simulink model "test"  (R2023b)
settings: Solver=VariableStepAuto  StartTime=0.0  StopTime=inf  RelTol=1e-3
values from neighbouring files (symbols this model uses):
  A = [0  1; 0  0]    [1-dof.mat]    (also in 2-dof.mat = [0 0 0 0 1 0 0 0 0 0 0 0 ... (16 elements, 4x4)]; ball_balancing_platform.mat = [0 0 0 0 0 0 0 0 0 0 0 0 ... (64 elements, 8x8)])
  B = [0 -0.1692]    [1-dof.mat]    (also in 2-dof.mat = [0  0; -0.253868468945  0; 0  0; 0  0.253868468945]; ball_balancing_platform.mat = [0 0 0 0 0 0 1 0 0 0 0 0 ... (16 elements, 8x2)])
  C = [1 0]    [1-dof.mat]    (also in 2-dof.mat = [1  0  0  0; 0  0  1  0]; ball_balancing_platform.mat = [1 0 0 0 0 1 0 0 0 0 1 0 ... (32 elements, 4x8)])
  D = 0    [1-dof.mat]    (also in 2-dof.mat = [0  0; 0  0]; ball_balancing_platform.mat = [0  0; 0  0; 0  0; 0  0])
libraries: mpclib x1, aerolibanimutils x1
settings Model: Creator=farhan  LastModifiedBy=farhan

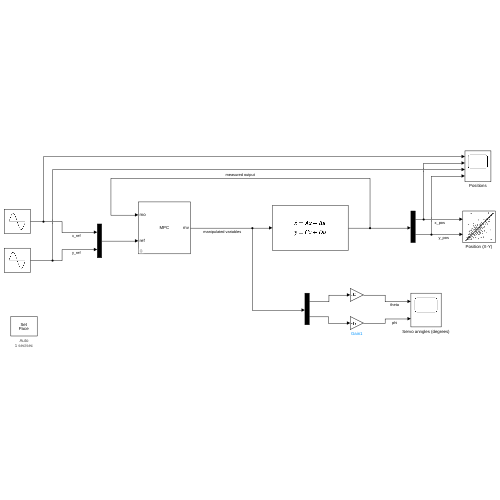
[thumbnail: Simulink's stored preview of the top-level diagram]
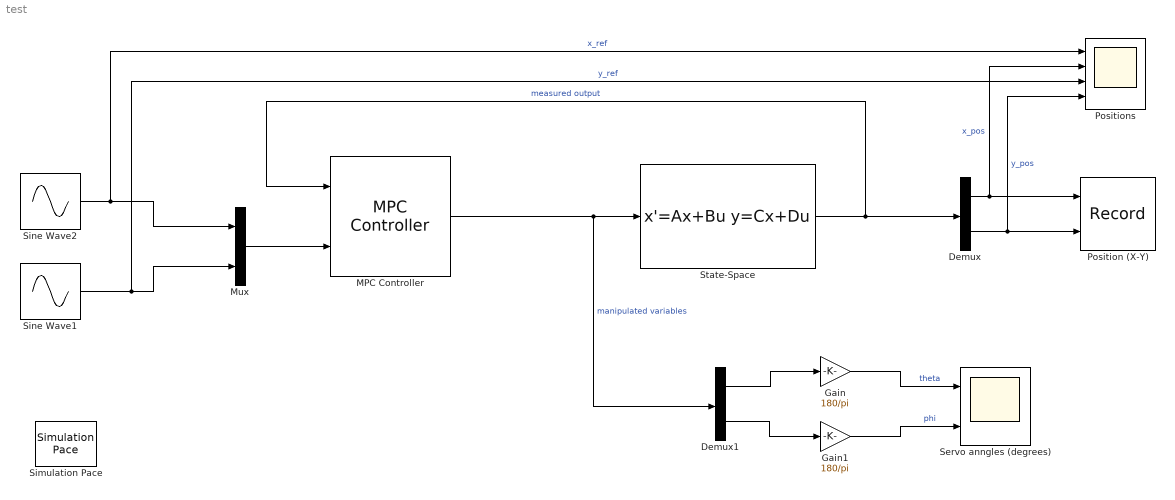
== system test ==
  Demux : Demux  Outputs=2
  Demux1 : Demux  Outputs=2
  Gain : Gain  Gain=180/pi
  Gain1 : Gain  Gain=180/pi
  MPC Controller : mpclib/MPC Controller  SCDEnableBlockLinearizationSpecification=on  mpcobj=mpc1  is_multiple=0  enable_value=0  return_u0=off  updateMPCinCallerWorkspace=on  md_inport=off  mv_inport=off  uref_inport=off  return_cost=off  return_mvseq=off  return_qpstatus=off  return_xseq=off  return_state=off  return_ovseq=off  state_inport=off  umin_inport=off  umax_inport=off  ymin_inport=off  ymax_inport=off  cc_inport=off  ywt_inport=off  uwt_inport=off  duwt_inport=off  rhoeps_inport=off  pm_inport=off  MaximumP=10  HorizonChoice=FixedHorizon  n_ts=0.1  n_p=7  n_mv=2  n_md=0  n_ud=0  n_mo=2  n_uo=0  BlockDataType=double  SampleTimeInherited=off  switch_inport=off
  Mux : Mux  Inputs=2
  Position (X-Y) : Record  FileSettingsInternal="{\"entries\":[{\"content\":{\"excelSettings\":{\"content\":{},\"type\":\"Streamout.ExcelSettings\"}},\"type\":\"Streamout.FileSettingStorage\",\"uuid\":\"\"}],\"packageUris\":[\"http:\\/\\/schema.mathworks.com\\/mf0\\/streamout_blocks\\/R2020a\"],\"version\":\"1.0\"}"  Layout=[1 1]  SignalsInternal="{\"entries\":[{\"content\":{\"signals\":[{\"content\":{\"blockPath\":[],\"dimensions\":[1],\"domain\":\"\",\"lineColor\":\"#fe330a\",\"port\":1,\"sid\":[\"\"],\"signalID\":130,\"signalName\":\"x_pos\"},\"type\":\"RecordBlkView.Signal\",\"uuid\":\"\"},{\"content\":{\"blockPath\":[],\"dimensions\":[1],\"domain\":\"\",\"lineColor\":\"#22b573\",\"port\":2,\"sid\":[\"\"],\"signalID\":134,\"signalName\":\"y_pos\"},\"type\":\"RecordBlkView.Signal\",\"uuid\":\"\"}]},\"type\":\"RecordBlkView.InputSignals\",\"uuid\":\"\"}],\"packageUris\":[\"http:\\/\\/schema.mathworks.com\\/mf0\\/streamout_blocks\\/R2020a\"],\"version\":\"1.0\"}"  VisualizationBindings="{\"xyplotplugin\":{\"info\":[{\"series\":[],\"subplotID\":1}]}}"  CompatibilityTag=XY
  Positions : Scope  NumInputPorts=4
  Servo anngles (degrees) : Scope  NumInputPorts=2
  Simulation Pace : aerolibanimutils/Simulation Pace  SimulationPace=1  SleepMode=Auto  OutputPaceError=off  SampleTime=1/30
  Sine Wave1 : Sin  Amplitude=0.15  Frequency=1.2  Phase=pi/2  SampleTime=0
  Sine Wave2 : Sin  Amplitude=0.15  Frequency=1.2  SampleTime=0
  State-Space : StateSpace  A=A  B=B  C=C  D=D  InitialCondition=0
  wires:
  MPC Controller/1 -> Demux1/1, State-Space/1  "manipulated variables"
  Mux/1 -> MPC Controller/2
  Sine Wave2/1 -> Mux/1, Positions/1  "x_ref"
  Sine Wave1/1 -> Mux/2, Positions/3  "y_ref"
  State-Space/1 -> Demux/1, MPC Controller/1  "measured output"
  Demux/1 -> Positions/2, Position (X-Y)/1  "x_pos"
  Demux/2 -> Positions/4, Position (X-Y)/2  "y_pos"
  Demux1/1 -> Gain/1
  Demux1/2 -> Gain1/1
  Gain/1 -> Servo anngles (degrees)/1  "theta"
  Gain1/1 -> Servo anngles (degrees)/2  "phi"
